simulink model "Helicopter_model"  (R2022a)
settings: Solver=ode45  StartTime=0.0  StopTime=100  MaxStep=.05  RelTol=1e-3  EnableMultiTasking=on
values from neighbouring files (symbols this model uses):
  gamma_q = 10    [Helicopter_data.m]
  gamma_qc = 10    [Helicopter_data.m]
  gamma_theta = 10    [Helicopter_data.m]
  theta = -0.01    [Helicopter_data.m]
libraries: cstblocks x1
settings Model: Creator=j.bordeneuve  LastModifiedBy=fades
settings SolverCC: AlgebraicLoopSolver=TrustRegion
settings DataIOCC: SaveFormat=Array  SignalLoggingSaveFormat=ModelDataLogs  ReturnWorkspaceOutputs=off  SignalLoggingName=sigsOut
settings OptimizationCC: InitFltsAndDblsToZero=on  LifeSpan=inf
settings DebuggingCC: SaveWithParameterizedLinksMsg=none  UnderspecifiedInitializationDetection=Classic  MergeDetectMultiDrivingBlocksExec=none  SignalResolutionControl=TryResolveAllWithWarning  MultiTaskDSMMsg=warning  MultiTaskCondExecSysMsg=none  UnconnectedInputMsg=warning  UnconnectedOutputMsg=warning  UnconnectedLineMsg=warning  AllowSymbolicDim=off  PregeneratedLibrarySubsystemCodeDiagnostic=none  SFUnexpectedBacktrackingDiag=warning  SFNoUnconditionalDefaultTransitionDiag=warning  SFExecutionAtInitializationDiag=none  SFMachineParentedDataDiag=warning  ArithmeticOperatorsInVariantConditions=warning
settings HardwareCC: ProdBitPerPointer=32  ProdBitPerSizeT=32  ProdBitPerPtrDiffT=32  ProdLargestAtomicFloat=None  ProdIntDivRoundTo=Undefined  ProdEndianess=Unspecified  ProdWordSize=32  ProdHWDeviceType=32-bit Generic  TargetUnknown=on
settings ModelReferenceCC: PropagateSignalLabelsOutOfModel=off
settings SFSimCC: SimUseLocalCustomCode=off  CustomCodeUndefinedFunction=UseInterfaceOnly
settings RTWCC: RTWUseLocalCustomCode=off  DLArmComputeVersion=19.05
settings CodeAppCC: StateflowObjectComments=on
settings GRTTargetCC: TargetFcnLib=ansi_tfl_tmw.mat  TargetLangStandard=C89/C90 (ANSI)  CombineOutputUpdateFcns=off  GRTInterface=on
settings ConfigComp: CovMetricSettings=dw  CovSaveCumulativeToWorkspaceVar=on  CovSaveSingleToWorkspaceVar=on  CovExternalEMLEnable=off

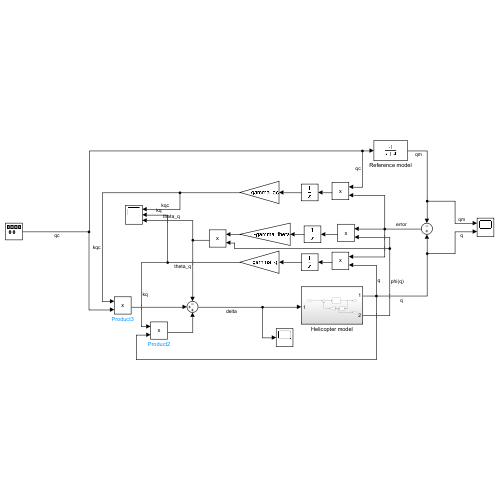
[thumbnail: Simulink's stored preview of the top-level diagram]
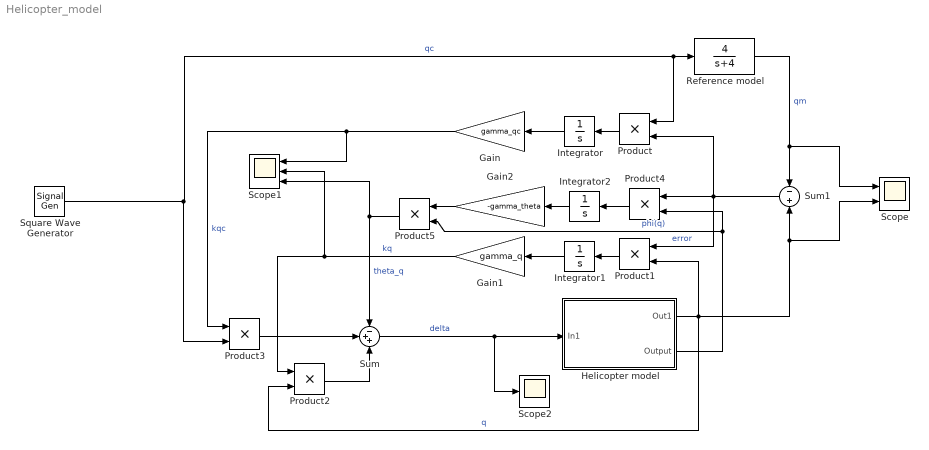
== system Helicopter_model ==
  Gain : Gain  Gain=gamma_qc
  Gain1 : Gain  Gain=gamma_q
  Gain2 : Gain  Gain=-gamma_theta
  Helicopter model : Subsystem
  Integrator : Integrator
  Integrator1 : Integrator
  Integrator2 : Integrator
  Product{,1..5} (6 alike) : Product
  Reference model : TransferFcn  Numerator=[4]  Denominator=[1 4]
  Scope : Scope  NumInputPorts=2
  Scope1 : Scope  NumInputPorts=3
  Scope2 : Scope
  Square Wave Generator : SignalGenerator  WaveForm=square  Frequency=0.05
  Sum : Sum  Inputs=-++
  Sum1 : Sum  Inputs=-+
  wires:
  Square Wave Generator/1 -> Product3/2, Product/1, Reference model/1  "qc"
  Helicopter model/1(Out1) -> Product2/2, Scope/2, Sum1/2, Product1/2  "q"
  Reference model/1 -> Sum1/1, Scope/1  "qm"
  Sum1/1 -> Product/2, Product4/1, Product1/1  "error"
  Product/1 -> Integrator/1
  Integrator/1 -> Gain/1
  Product1/1 -> Integrator1/1
  Integrator1/1 -> Gain1/1
  Sum/1 -> Scope2/1, Helicopter model/1(In1)  "delta"
  Gain/1 -> Scope1/1, Product3/1  "kqc"
  Product3/1 -> Sum/2
  Gain1/1 -> Scope1/2, Product2/1  "kq"
  Product2/1 -> Sum/3
  Product5/1 -> Scope1/3, Sum/1  "theta_q"
  Gain2/1 -> Product5/1
  Product4/1 -> Integrator2/1
  Integrator2/1 -> Gain2/1
  Helicopter model/2(Output) -> Product5/2, Product4/2  "phi(q)"

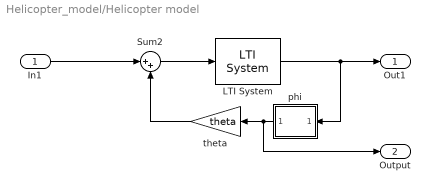
== system Helicopter_model/Helicopter model ==
  In1 : Inport
  LTI System : cstblocks/LTI System  sys=heli_lin  IC=[]
  Sum2 : Sum  Inputs=|++
  phi : Subsystem
  theta : Gain  Gain=theta
  Out1 : Outport
  Output : Outport  Port=2
  wires:
  Sum2/1 -> LTI System/1
  theta/1 -> Sum2/2
  phi/1(Output) -> Output/1, theta/1
  In1/1 -> Sum2/1
  LTI System/1 -> Out1/1, phi/1(In1)

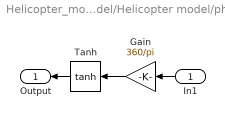
== system Helicopter_model/Helicopter model/phi ==
  In1 : Inport
  Gain : Gain  Gain=360/pi
  Tanh : Trigonometry  Operator=tanh
  Output : Outport
  wires:
  Tanh/1 -> Output/1
  In1/1 -> Gain/1
  Gain/1 -> Tanh/1
